simulink model "ctrl_custom"  (R2016b)
settings: Solver=ode3  StartTime=0.0  StopTime=inf  FixedStep=0.01  RelTol=1e-3  EnableMultiTasking=on
values from neighbouring files (symbols this model uses):
  C = [C1;C2;C3;C4;C5;C6]    [initfile.m]
  D = 3.0/100    (= 0.03)    [initfile.m]
  eps_c = 5    [initfile.m]
  epsilon = 0.5    [initfile.m]
  hd = c2d(H1,0.01,'foh')    [initfile.m]
  hd2 = c2d(H2,0.01,'zoh')    [initfile.m]
  I_s = 25000 /747225    (= 0.0334571246947)    [initfile.m]
  k_cc = 1    [initfile.m]
  K_omega = 0.3    [initfile.m]
  K_q1f = 0.0113    [initfile.m]
  K_q1r = K_q1f    (= 0.0113)    [initfile.m]
  K_q2f = 0.0117    [initfile.m]
  K_q2r = K_q2f    (= 0.0117)    [initfile.m]
  K_q3f = 0.0113    [initfile.m]
  K_q3r = K_q3f    (= 0.0113)    [initfile.m]
  K_q4f = 0.0169    [initfile.m]
  K_q4r = K_q4f    (= 0.0169)    [initfile.m]
  K_q5f = 0.0144    [initfile.m]
  K_q5r = K_q5f    (= 0.0144)    [initfile.m]
  K_q6f = 0.0168    [initfile.m]
  K_q6r = K_q6f    (= 0.0168)    [initfile.m]
  K_T1f = 0.3763    [initfile.m]
  K_T1r = K_T1f    (= 0.3763)    [initfile.m]
  K_T2f = 0.3901    [initfile.m]
  K_T2r = K_T2f    (= 0.3901)    [initfile.m]
  K_T3f = 0.3776    [initfile.m]
  K_T3r = K_T3f    (= 0.3776)    [initfile.m]
  K_T4f = 0.5641    [initfile.m]
  K_T4r = K_T4f    (= 0.5641)    [initfile.m]
  K_T5f = 0.4799    [initfile.m]
  K_T5r = K_T5f    (= 0.4799)    [initfile.m]
  K_T6f = 0.5588    [initfile.m]
  K_T6r = K_T6f    (= 0.5588)    [initfile.m]
  Kp = 3.3    [initfile.m]
  Max_Acceleration = 5    [initfile.m]
  Max_rotation = 12*sqrt(lambda)    [initfile.m]
  Max_thrust = 1.5    [initfile.m]
  Min_thrust = -0.8    [initfile.m]
  n_c = 5    [initfile.m]
  n_max = 152    [initfile.m]
  p_cc = 0.5    [initfile.m]
  pwm_thr1_backward = coeffvalues(ForceToPWM)    [initfile.m]
  pwm_thr1_forward = coeffvalues(ForceToPWM)    [initfile.m]
  pwm_thr2_backward = coeffvalues(ForceToPWM)    [initfile.m]
  pwm_thr2_forward = coeffvalues(ForceToPWM)    [initfile.m]
  pwm_thr3_backward = coeffvalues(ForceToPWM)    [initfile.m]
  pwm_thr3_forward = coeffvalues(ForceToPWM)    [initfile.m]
  pwm_thr4_backward = coeffvalues(ForceToPWM)    [initfile.m]
  pwm_thr4_forward = coeffvalues(ForceToPWM)    [initfile.m]
  pwm_thr5_backward = coeffvalues(ForceToPWM)    [initfile.m]
  pwm_thr5_forward = coeffvalues(ForceToPWM)    [initfile.m]
  pwm_thr6_backward = coeffvalues(ForceToPWM)    [initfile.m]
  pwm_thr6_forward = coeffvalues(ForceToPWM)    [initfile.m]
  Q_f0 = 0.3    [initfile.m]
  r_cc = 4    [initfile.m]
  Rho = Rho_m    (= 1000)    [initfile.m]
undefined symbols (not defined in the file or in its folder): DiscIntNeverNeededParam, Q_max, Thruster
libraries: dspmtrx3 x9, marine_gnc x8, simulink x7, simulink_extras x3
(part 6 of 6)

== matlab function ctrl_custom/MATLAB Function ==
  data: thrust_actual input; commanded_tau output; alpha_actual input; PosX input; PosY input
function commanded_tau   = fcn(thrust_actual,alpha_actual,PosX,PosY)
%#codegen

Alpha_surge =[cosd(alpha_actual(1)) cosd(alpha_actual(2)) cosd(alpha_actual(3)) cosd(alpha_actual(4)) cosd(alpha_actual(5)) cosd(alpha_actual(6))];  
Alpha_sway = [sind(alpha_actual(1)) sind(alpha_actual(2)) sind(alpha_actual(3)) sind(alpha_actual(4)) sind(alpha_actual(5)) sind(alpha_actual(6))];
Alpha_yaw = [sind(alpha_actual(1))*PosX(1)-cosd(alpha_actual(1))*PosY(1) sind(alpha_actual(2))*PosX(2)-cosd(alpha_actual(2))*PosY(2) ...
             sind(alpha_actual(3))*PosX(3)-cosd(alpha_actual(3))*PosY(3) sind(alpha_actual(4))*PosX(4)-cosd(alpha_actual(4))*PosY(4) ...
             sind(alpha_actual(5))*PosX(5)-cosd(alpha_actual(5))*PosY(5) sind(alpha_actual(6))*PosX(6)-cosd(alpha_actual(6))*PosY(6)];

commanded_tau = [Alpha_surge;Alpha_sway;Alpha_yaw]*thrust_actual;

== matlab function ctrl_custom/Thruster control /Thrust and Shaft speed mapped to PWM/MATLAB Function5 ==
  data: Tc_in1 input; signal input; Tc_out output; Tc_in2 input
function Tc_out = fcn(Tc_in1,signal,Tc_in2)
%#codegen

if signal >= 0
    Tc_out = Tc_in1;
else %signal < 0
    Tc_out = Tc_in2;
end

== matlab function ctrl_custom/Thruster control /Thruster 3/Thruster control/Core controller/Core controller: Torque,Power and Combined Torque//Power ==
  data: Qcq output; Qcp output; k_cc input; p_cc input; r_cc input; n input; Qcc output; K_t0 input; K_q0 input; D input; Tr input; rho input; eps_c input; K_t0r input; K_q0r input
function [Qcq,Qcp,Qcc]= CoreControl(k_cc,p_cc,r_cc,n,K_t0,K_q0,D,Tr,rho,eps_c,K_t0r,K_q0r)
%#codegen

lambda_c = 0.5+0.5*tanh(eps_c*n/5);
K_TC = K_t0*lambda_c+(1-lambda_c)*K_t0r;
K_QC = K_q0*lambda_c+(1-lambda_c)*K_q0r;
Qcq = (K_QC/K_TC)*D*Tr;
if n == 0
    Qcp = 0;
else
Qcp = sign(Tr)*K_QC*(abs(Tr)^(3/2))/(sqrt(rho)*D*K_TC^(3/2)*abs(n));
end
alpha_c = exp(-k_cc*abs(p_cc*n)^r_cc);

Qcc = alpha_c*Qcq + (1-alpha_c)*Qcp;

== matlab function ctrl_custom/Thruster control /Thruster 3/Thruster control/MATLAB Function ==
  data: Td input; n_d output; K_t0 input; K_t0r input; rho input; D input; eps_c input; n_c input; n_r input; T_r output
function [n_d,T_r]  = ReferenceGenerator(Td,K_t0,K_t0r,rho,D,eps_c,n_c,n_r)
%#codegen


n_d = sign(Td)*sqrt((abs(Td))/(rho*D^4*K_t0));

lambda_c = 0.5+0.5*tanh(eps_c*n_d/5); % Smooth switching between positive and negative thrust
K_TC = K_t0*lambda_c+(1-lambda_c)*K_t0r;

T_r = sign(n_r)*K_TC*rho*D^4*n_r^2;

== matlab function ctrl_custom/Thruster control /Thrust and Shaft speed mapped to PWM/MATLAB Function ==
  data: input input; output output; control input; speedcontrol input
function output = fcn(input,control,speedcontrol)
%#codegen
if control == 1
output = [input(1) speedcontrol(1) input(3) speedcontrol(2) input(5) speedcontrol(3) input(7) speedcontrol(4) input(9) speedcontrol(5) input(11) speedcontrol(6)]';
%     output = [input(1) input(2) input(3) input(4) input(5) input(6) input(7) input(8) input(9) input(10) input(11) input(12)]';

else
    output = [input(1) input(2) input(3) input(4) input(5) input(6) input(7) input(8) input(9) input(10) input(11) input(12)]';

end

== matlab function ctrl_custom/Thruster control /Thrust and Shaft speed mapped to PWM/MATLAB Function6 ==
  data: Tc_in1 input; signal input; Tc_out output; Tc_in2 input
function Tc_out = fcn(Tc_in1,signal,Tc_in2)
%#codegen

if signal >= 0
    Tc_out = Tc_in1;
else %signal < 0
    Tc_out = Tc_in2;
end

== matlab function ctrl_custom/Thruster control /Thruster 3/Thruster control/Supervisor ==
  data: control input; input input; n input; u output
function u = fcn(control,input,n)
u = 1;
if control == 1
if input == 1
    u = 1;
elseif input == 2
    u = 2;
elseif input == 3 && n > 0 || input == 3 && n < 0
    u = 3;
elseif input == 4 || input == 3 && n == 0
    u = 4;
else 
    u = 5;
end
end

if control == 2
if input == 1
    u = 1;
elseif input == 2
    u = 2;
elseif input == 3 && n > 0 || input == 3 && n < 0
    u = 3;
elseif input == 4 || input == 3 && n == 0
    u = 4;
else 
    u = 5;
end
end

if control == 3
if input == 1
    u = 1;
elseif input == 2
    u = 2;
elseif input == 3 && n > 0 || input == 3 && n < 0
    u = 3;
elseif input == 4 || input == 3 && n == 0
    u = 4;
else 
    u = 5;
end
end

if control == 4
if input == 1
    u = 1;
elseif input == 2
    u = 2;
elseif input == 3 && n > 0 || input == 3 && n < 0
    u = 3;
elseif input == 4 || input == 3 && n == 0
    u = 4;
else 
    u = 5;
end
end

if control == 5
if input == 1
    u = 1;
elseif input == 2
    u = 2;
elseif input == 3 && n > 0 || input == 3 && n < 0
    u = 3;
elseif input == 4 || input == 3 && n == 0
    u = 4;
else 
    u = 5;
end
end

== matlab function ctrl_custom/Thruster control /Thruster 4/Propeller Hydrodynamics/Actual Force and Torque ==
  data: Ta output; n input; Qa output; Kq input; Kt input; Ktr input; Kqr input; Rho input; D input; eps_c input; env input
function [Ta,Qa]= ActualForces(n,Kq,Kt,Ktr,Kqr,Rho,D,eps_c,env)
%#codegen
lambda_c = 0.5+0.5*tanh(eps_c*n/5); % Smooth switching between positive and negative thrust. 5 makes switch happen between -5 and 5
K_TC = Kt*lambda_c+(1-lambda_c)*Ktr;
K_QC = Kq*lambda_c+(1-lambda_c)*Kqr;

Ta = sign(n)*K_TC*Rho*(D^4)*n^2-env;
Qa = sign(n)*K_QC*Rho*(D^5)*n^2-env;

== matlab function ctrl_custom/Thruster control /Thruster 4/Thruster control/Core controller/Core controller: Torque,Power and Combined Torque//Power ==
  data: Qcq output; Qcp output; k_cc input; p_cc input; r_cc input; n input; Qcc output; K_t0 input; K_q0 input; D input; Tr input; rho input; eps_c input; K_t0r input; K_q0r input
function [Qcq,Qcp,Qcc]= CoreControl(k_cc,p_cc,r_cc,n,K_t0,K_q0,D,Tr,rho,eps_c,K_t0r,K_q0r)
%#codegen

lambda_c = 0.5+0.5*tanh(eps_c*n/5);
K_TC = K_t0*lambda_c+(1-lambda_c)*K_t0r;
K_QC = K_q0*lambda_c+(1-lambda_c)*K_q0r;
Qcq = (K_QC/K_TC)*D*Tr;
if n == 0
    Qcp = 0;
else
Qcp = sign(Tr)*K_QC*(abs(Tr)^(3/2))/(sqrt(rho)*D*K_TC^(3/2)*abs(n));
end
alpha_c = exp(-k_cc*abs(p_cc*n)^r_cc);

Qcc = alpha_c*Qcq + (1-alpha_c)*Qcp;

== matlab function ctrl_custom/Thruster control /Thruster 4/Thruster control/MATLAB Function ==
  data: Td input; n_d output; K_t0 input; K_t0r input; rho input; D input; eps_c input; n_c input; n_r input; T_r output
function [n_d,T_r]  = ReferenceGenerator(Td,K_t0,K_t0r,rho,D,eps_c,n_c,n_r)
%#codegen


n_d = sign(Td)*sqrt((abs(Td))/(rho*D^4*K_t0));

lambda_c = 0.5+0.5*tanh(eps_c*n_d/5); % Smooth switching between positive and negative thrust
K_TC = K_t0*lambda_c+(1-lambda_c)*K_t0r;

T_r = sign(n_r)*K_TC*rho*D^4*n_r^2;

== matlab function ctrl_custom/Thruster control /Thruster 4/Thruster control/Supervisor ==
  data: control input; input input; n input; u output
function u = fcn(control,input,n)
u = 1;
if control == 1
if input == 1
    u = 1;
elseif input == 2
    u = 2;
elseif input == 3 && n > 0 || input == 3 && n < 0
    u = 3;
elseif input == 4 || input == 3 && n == 0
    u = 4;
else 
    u = 5;
end
end

if control == 2
if input == 1
    u = 1;
elseif input == 2
    u = 2;
elseif input == 3 && n > 0 || input == 3 && n < 0
    u = 3;
elseif input == 4 || input == 3 && n == 0
    u = 4;
else 
    u = 5;
end
end

if control == 3
if input == 1
    u = 1;
elseif input == 2
    u = 2;
elseif input == 3 && n > 0 || input == 3 && n < 0
    u = 3;
elseif input == 4 || input == 3 && n == 0
    u = 4;
else 
    u = 5;
end
end

if control == 4
if input == 1
    u = 1;
elseif input == 2
    u = 2;
elseif input == 3 && n > 0 || input == 3 && n < 0
    u = 3;
elseif input == 4 || input == 3 && n == 0
    u = 4;
else 
    u = 5;
end
end

if control == 5
if input == 1
    u = 1;
elseif input == 2
    u = 2;
elseif input == 3 && n > 0 || input == 3 && n < 0
    u = 3;
elseif input == 4 || input == 3 && n == 0
    u = 4;
else 
    u = 5;
end
end

== matlab function ctrl_custom/Thruster control /Thruster 5/Propeller Hydrodynamics/Actual Force and Torque ==
  data: Ta output; n input; Qa output; Kq input; Kt input; Ktr input; Kqr input; Rho input; D input; eps_c input; env input
function [Ta,Qa]= ActualForces(n,Kq,Kt,Ktr,Kqr,Rho,D,eps_c,env)
%#codegen
lambda_c = 0.5+0.5*tanh(eps_c*n/5); % Smooth switching between positive and negative thrust. 5 makes switch happen between -5 and 5
K_TC = Kt*lambda_c+(1-lambda_c)*Ktr;
K_QC = Kq*lambda_c+(1-lambda_c)*Kqr;

Ta = sign(n)*K_TC*Rho*(D^4)*n^2-env;
Qa = sign(n)*K_QC*Rho*(D^5)*n^2-env;

== matlab function ctrl_custom/Thruster control /Thruster 5/Thruster control/Core controller/Core controller: Torque,Power and Combined Torque//Power ==
  data: Qcq output; Qcp output; k_cc input; p_cc input; r_cc input; n input; Qcc output; K_t0 input; K_q0 input; D input; Tr input; rho input; eps_c input; K_t0r input; K_q0r input
function [Qcq,Qcp,Qcc]= CoreControl(k_cc,p_cc,r_cc,n,K_t0,K_q0,D,Tr,rho,eps_c,K_t0r,K_q0r)
%#codegen

lambda_c = 0.5+0.5*tanh(eps_c*n/5);
K_TC = K_t0*lambda_c+(1-lambda_c)*K_t0r;
K_QC = K_q0*lambda_c+(1-lambda_c)*K_q0r;
Qcq = (K_QC/K_TC)*D*Tr;
if n == 0
    Qcp = 0;
else
Qcp = sign(Tr)*K_QC*(abs(Tr)^(3/2))/(sqrt(rho)*D*K_TC^(3/2)*abs(n));
end
alpha_c = exp(-k_cc*abs(p_cc*n)^r_cc);

Qcc = alpha_c*Qcq + (1-alpha_c)*Qcp;

== matlab function ctrl_custom/Thruster control /Thruster 5/Thruster control/MATLAB Function ==
  data: Td input; n_d output; K_t0 input; K_t0r input; rho input; D input; eps_c input; n_c input; n_r input; T_r output
function [n_d,T_r]  = ReferenceGenerator(Td,K_t0,K_t0r,rho,D,eps_c,n_c,n_r)
%#codegen


n_d = sign(Td)*sqrt((abs(Td))/(rho*D^4*K_t0));

lambda_c = 0.5+0.5*tanh(eps_c*n_d/5); % Smooth switching between positive and negative thrust
K_TC = K_t0*lambda_c+(1-lambda_c)*K_t0r;

T_r = sign(n_r)*K_TC*rho*D^4*n_r^2;

== matlab function ctrl_custom/Thruster control /Thruster 5/Thruster control/Supervisor ==
  data: control input; input input; n input; u output
function u = fcn(control,input,n)
u = 1;
if control == 1
if input == 1
    u = 1;
elseif input == 2
    u = 2;
elseif input == 3 && n > 0 || input == 3 && n < 0
    u = 3;
elseif input == 4 || input == 3 && n == 0
    u = 4;
else 
    u = 5;
end
end

if control == 2
if input == 1
    u = 1;
elseif input == 2
    u = 2;
elseif input == 3 && n > 0 || input == 3 && n < 0
    u = 3;
elseif input == 4 || input == 3 && n == 0
    u = 4;
else 
    u = 5;
end
end

if control == 3
if input == 1
    u = 1;
elseif input == 2
    u = 2;
elseif input == 3 && n > 0 || input == 3 && n < 0
    u = 3;
elseif input == 4 || input == 3 && n == 0
    u = 4;
else 
    u = 5;
end
end

if control == 4
if input == 1
    u = 1;
elseif input == 2
    u = 2;
elseif input == 3 && n > 0 || input == 3 && n < 0
    u = 3;
elseif input == 4 || input == 3 && n == 0
    u = 4;
else 
    u = 5;
end
end

if control == 5
if input == 1
    u = 1;
elseif input == 2
    u = 2;
elseif input == 3 && n > 0 || input == 3 && n < 0
    u = 3;
elseif input == 4 || input == 3 && n == 0
    u = 4;
else 
    u = 5;
end
end

== matlab function ctrl_custom/Thruster control /Thruster 6/Propeller Hydrodynamics/Actual Force and Torque ==
  data: Ta output; n input; Qa output; Kq input; Kt input; Ktr input; Kqr input; Rho input; D input; eps_c input; env input
function [Ta,Qa]= ActualForces(n,Kq,Kt,Ktr,Kqr,Rho,D,eps_c,env)
%#codegen
lambda_c = 0.5+0.5*tanh(eps_c*n/5); % Smooth switching between positive and negative thrust. 5 makes switch happen between -5 and 5
K_TC = Kt*lambda_c+(1-lambda_c)*Ktr;
K_QC = Kq*lambda_c+(1-lambda_c)*Kqr;

Ta = sign(n)*K_TC*Rho*(D^4)*n^2-env;
Qa = sign(n)*K_QC*Rho*(D^5)*n^2-env;

== matlab function ctrl_custom/Thruster control /Thruster 6/Thruster control/Core controller/Core controller: Torque,Power and Combined Torque//Power ==
  data: Qcq output; Qcp output; k_cc input; p_cc input; r_cc input; n input; Qcc output; K_t0 input; K_q0 input; D input; Tr input; rho input; eps_c input; K_t0r input; K_q0r input
function [Qcq,Qcp,Qcc]= CoreControl(k_cc,p_cc,r_cc,n,K_t0,K_q0,D,Tr,rho,eps_c,K_t0r,K_q0r)
%#codegen

lambda_c = 0.5+0.5*tanh(eps_c*n/5);
K_TC = K_t0*lambda_c+(1-lambda_c)*K_t0r;
K_QC = K_q0*lambda_c+(1-lambda_c)*K_q0r;
Qcq = (K_QC/K_TC)*D*Tr;
if n == 0
    Qcp = 0;
else
Qcp = sign(Tr)*K_QC*(abs(Tr)^(3/2))/(sqrt(rho)*D*K_TC^(3/2)*abs(n));
end
alpha_c = exp(-k_cc*abs(p_cc*n)^r_cc);

Qcc = alpha_c*Qcq + (1-alpha_c)*Qcp;

== matlab function ctrl_custom/Thruster control /Thruster 6/Thruster control/MATLAB Function ==
  data: Td input; n_d output; K_t0 input; K_t0r input; rho input; D input; eps_c input; n_c input; n_r input; T_r output
function [n_d,T_r]  = ReferenceGenerator(Td,K_t0,K_t0r,rho,D,eps_c,n_c,n_r)
%#codegen


n_d = sign(Td)*sqrt((abs(Td))/(rho*D^4*K_t0));

lambda_c = 0.5+0.5*tanh(eps_c*n_d/27); % Smooth switching between positive and negative thrust
K_TC = K_t0*lambda_c+(1-lambda_c)*K_t0r;

T_r = sign(n_r)*K_TC*rho*D^4*n_r^2;

== matlab function ctrl_custom/Thruster control /Thruster 6/Thruster control/Supervisor ==
  data: control input; input input; n input; u output
function u = fcn(control,input,n)
u = 1;
if control == 1
if input == 1
    u = 1;
elseif input == 2
    u = 2;
elseif input == 3 && n > 0 || input == 3 && n < 0
    u = 3;
elseif input == 4 || input == 3 && n == 0
    u = 4;
else 
    u = 5;
end
end

if control == 2
if input == 1
    u = 1;
elseif input == 2
    u = 2;
elseif input == 3 && n > 0 || input == 3 && n < 0
    u = 3;
elseif input == 4 || input == 3 && n == 0
    u = 4;
else 
    u = 5;
end
end

if control == 3
if input == 1
    u = 1;
elseif input == 2
    u = 2;
elseif input == 3 && n > 0 || input == 3 && n < 0
    u = 3;
elseif input == 4 || input == 3 && n == 0
    u = 4;
else 
    u = 5;
end
end

if control == 4
if input == 1
    u = 1;
elseif input == 2
    u = 2;
elseif input == 3 && n > 0 || input == 3 && n < 0
    u = 3;
elseif input == 4 || input == 3 && n == 0
    u = 4;
else 
    u = 5;
end
end

if control == 5
if input == 1
    u = 1;
elseif input == 2
    u = 2;
elseif input == 3 && n > 0 || input == 3 && n < 0
    u = 3;
elseif input == 4 || input == 3 && n == 0
    u = 4;
else 
    u = 5;
end
end

== matlab function ctrl_custom/Nonlinear Passisve Observer/C(nu)*nu ==
  data: nu_hat input; C_nl output
function C_nl = fcn(nu_hat)
%#codegen
u = nu_hat(1);
v = nu_hat(2);
r = nu_hat(3);

%% MATRICES
m    = 127.92;   x_g = 0; %0.0432;

%% Added mass
X_ud  =   3.262;	Y_vd =      28.89;		Y_rd =      0.525;

%% Correolis matrix
c_13 = -(m-Y_vd)*v-(m*x_g-Y_rd)*r;
c_23 = (m-X_ud)*u;

C    = [0     0     c_13
        0     0     c_23
        -c_13 -c_23 0   ];

    
C_NL = C;

C_nl =C_NL*nu_hat;

== matlab function ctrl_custom/Nonlinear Passisve Observer/D(nu)*nu ==
  data: nu_hat input; D_nl output
function D_nl = fcn(nu_hat)
%#codegen
u = nu_hat(1);
v = nu_hat(2);
r = nu_hat(3);

%% DAMPING 

% Surge:
% Based on fitting of towing data from -0.8 < u < 0.8 m/s
X_u     = -2.332;
X_uu	=  0;
X_uuu	= -8.557;

% Sway:
% Based on fitting of towing data from -0.45 < u < 0.45 m/s
Y_v 	= -4.673;
Y_vv	=  0.3976;
Y_vvv	= -313.3;

% Yaw:
% Based on fitting of towing data from -8 < u < 8 deg/s
% The fitting range is limited. Towing should be performed for higher
% velocities.
N_r		= -0.01675;
N_rr	= -0.01148;
N_rrr	= -0.0003578;

% Y_vvv og N_rrr er fra curvefitting uten minus, men ser ut til å fungere
% med minus. 
                           N_v		= 0;                Y_r	    =  -7.250; 
                           N_vv	    = -0.2088;          Y_rr	=  -3.450;
                           N_vvv	= 0;                Y_rrr	=  0;
						
						   Y_rv	    = -0.805;			Y_vr	=  -0.845; 

						   N_rv	    = 0.08;             N_vr	= 0.08;
                           
%% Assembly of the damping matrix
d_11 = X_u + X_uu*abs(u) + X_uuu*u^2;
d_22 = Y_v + Y_vv*abs(v) + Y_vvv*v^2;
d_33 = N_r + N_rr*abs(r) + N_rrr*r^2;

d_23 = 0; % Y_r + Y_rr*abs(r) + Y_rrr*r^2 + Y_vr*abs(v); Not verified, temporarily disabled
d_32 = 0; % N_v + N_vv*abs(v) + N_vvv*v^2 + N_rv*abs(r); Not verified, temporarily disabled

D    = - [d_11 0    0
          0    d_22 d_23
          0    d_32 d_33];


D_NL = D;

D_nl =D_NL*nu_hat;
